simulink model "SMC0"  (R2018b)
settings: Solver=VariableStepAuto  StartTime=0.0  StopTime=20  RelTol=1e-3  EnableMultiTasking=on
settings Model: Creator=omid_zandi  LastModifiedBy=Arash
settings OptimizationCC: LifeSpan=inf
settings DebuggingCC: SFUnexpectedBacktrackingDiag=warning  SFNoUnconditionalDefaultTransitionDiag=warning
settings SFSimCC: SimUseLocalCustomCode=off
settings RTWCC: RTWUseLocalCustomCode=off
settings CodeAppCC: StateflowObjectComments=on
settings GRTTargetCC: TargetLangStandard=C89/C90 (ANSI)  GeneratePreprocessorConditionals=Disable all
settings ConfigComp: CovMetricSettings=dw  CovHtmlReporting=on  CovSaveCumulativeToWorkspaceVar=on  CovSaveSingleToWorkspaceVar=on  CovExternalEMLEnable=off

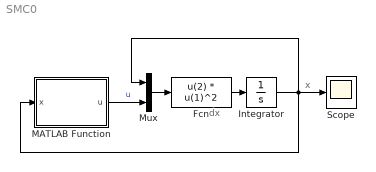
== system SMC0 ==
  note: dx
  note: x
  Fcn : Fcn  Expr=u(2) * u(1)^2
  Integrator : Integrator  InitialCondition=randn(1)*10
  MATLAB Function : MATLAB Function  TreatAsAtomicUnit=on
  Mux : Mux  Inputs=2
  Scope : Scope
  wires:
  Integrator/1 -> Mux/1, MATLAB Function/1(x), Scope/1
  Mux/1 -> Fcn/1
  Fcn/1 -> Integrator/1
  MATLAB Function/1(u) -> Mux/2  "u"

== matlab function SMC0/MATLAB Function ==
  data: x input; u output
function u = fcn(x)

u = -10 * sign(x);
